simulink model "manning_test_merge_nonlinear"  (R2022b)
settings: Solver=VariableStepAuto  StartTime=0.0  StopTime=5*N  RelTol=1e-3
libraries: cstblocks x2
settings Model: Creator=chuan  LastModifiedBy=chuan

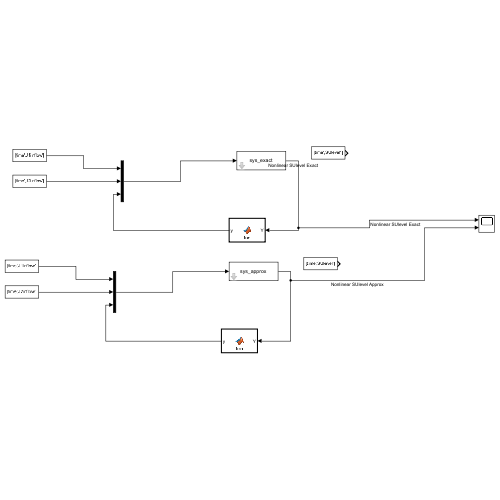
[thumbnail: Simulink's stored preview of the top-level diagram]
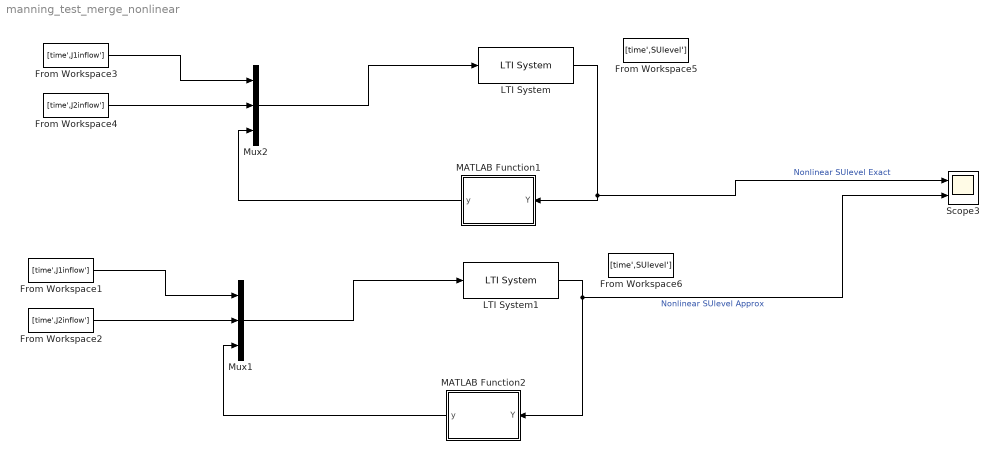
== system manning_test_merge_nonlinear ==
  From Workspace1 : FromWorkspace  VariableName=[time',J1inflow']
  From Workspace2 : FromWorkspace  VariableName=[time',J2inflow']
  From Workspace3 : FromWorkspace  VariableName=[time',J1inflow']
  From Workspace4 : FromWorkspace  VariableName=[time',J2inflow']
  From Workspace5 : FromWorkspace  VariableName=[time',SUlevel']
  From Workspace6 : FromWorkspace  VariableName=[time',SUlevel']
  LTI System : cstblocks/LTI System  sys=sys_exact  IC=[]
  LTI System1 : cstblocks/LTI System  sys=sys_approx  IC=[]
  MATLAB Function1 : MATLAB Function  TreatAsAtomicUnit=on
  MATLAB Function2 : MATLAB Function  TreatAsAtomicUnit=on
  Mux1 : Mux  Inputs=3
  Mux2 : Mux  Inputs=3
  Scope3 : Scope  NumInputPorts=2
  wires:
  Mux2/1 -> LTI System/1
  LTI System/1 -> Scope3/1, MATLAB Function1/1(Y)  "Nonlinear SUlevel Exact"
  MATLAB Function1/1(y) -> Mux2/3
  From Workspace3/1 -> Mux2/1
  From Workspace4/1 -> Mux2/2
  From Workspace1/1 -> Mux1/1
  From Workspace2/1 -> Mux1/2
  MATLAB Function2/1(y) -> Mux1/3
  LTI System1/1 -> Scope3/2, MATLAB Function2/1(Y)  "Nonlinear SUlevel Approx"
  Mux1/1 -> LTI System1/1

== matlab function manning_test_merge_nonlinear/MATLAB Function1 ==
  data: Y input; y output
function y = fcn(Y)
Cd = 0.65;
A0 = 144;
g = 9.81;
Z0 = 0;
Yfull = 12;
H_star = Z0 + Yfull;

Y = max(Y,0);
H1 = Y + Z0;

if H1 >= H_star
    He = H1 - (Z0 + Yfull/2);
    y = Cd*A0*sqrt(2*g*He);
else
    CwL = (Cd*A0*sqrt(g))/(Yfull);
    y = CwL*(H1-Z0)^(1.5);
end

== matlab function manning_test_merge_nonlinear/MATLAB Function2 ==
  data: Y input; y output
function y = fcn(Y)
Cd = 0.65;
A0 = 144;
g = 9.81;
Z0 = 0;
Yfull = 12;
H_star = Z0 + Yfull;

Y = max(Y,0);
H1 = Y + Z0;

if H1 >= H_star
    He = H1 - (Z0 + Yfull/2);
    y = Cd*A0*sqrt(2*g*He);
else
    CwL = (Cd*A0*sqrt(g))/(Yfull);
    y = CwL*(H1-Z0)^(1.5);
end
